simulink library "xpcrealtimedeviceslib"  (Simulink 6.0)
settings: Solver=ode45  SolverMode=SingleTasking  StartTime=0.0  StopTime=10.0  RelTol=1e-3
values from neighbouring files (symbols this model uses):
  baseDec = hex2dec(base(3:end))    [maddiamondmm.m]    (also in maddiamondmm32.m; maddiamondmm32frame.m; maddsmm16at.m; madprometheus.m)
undefined symbols (not defined in the file or in its folder): madrtddm64x0, madrtddm7420, mdartddm6430, mdartddm64x0, mdiortddm64x0, mdiortddm7420, mdirtddm6814, mdortddm6814, mencrtddm6814, misa8255, mpwmrtddm6816, mrtddm6604
libraries: xpcmeasurementcomputinglib x6
settings Model: Creator=adowd  LastModifiedBy=gweast
settings DataIOCC: SignalLoggingName=logsOut
settings OptimizationCC: BooleanDataType=off
settings DebuggingCC: CheckExecutionContextPreStartOutputMsg=on  CheckExecutionContextRuntimeOutputMsg=on  SolverPrmCheckMsg=none
settings HardwareCC: TargetUnknown=on
settings GRTTargetCC: UtilityFuncGeneration=Automatic  LifeSpan=inf
settings SFSimCC: SFSimApplyToAllLibs=on  SFSimBuildMode=Incremental

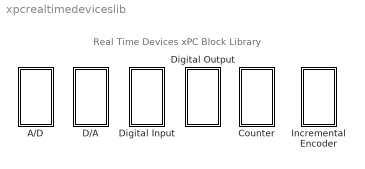
== system xpcrealtimedeviceslib ==
  note: Real Time Devices xPC Block Library
  A/D : Subsystem  EnableExecutionContextPropagation=on
  Counter : Subsystem  EnableExecutionContextPropagation=on
  D/A : Subsystem  EnableExecutionContextPropagation=on
  Digital Input : Subsystem  EnableExecutionContextPropagation=on
  Digital Output : Subsystem  EnableExecutionContextPropagation=on
  Incremental Encoder : Subsystem  EnableExecutionContextPropagation=on

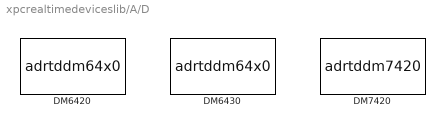
== system xpcrealtimedeviceslib/A/D ==
  "DM6420 " : S-Function  InitFcn=madrtddm64x0(1);  FunctionName=adrtddm64x0  Parameters=channel, coupling, range, gain, ts, baseAddr, boardType  mask(adrtddm6420){channelin=[1], couplingin=[1], rangein=[-10], gainin=[1], ts=0.001, baseAddr=0x300}
      mask prompts: channelin "Channel vector:"; couplingin "Input coupling vector:"; rangein "Range vector:"; gainin "Gain vector:"; ts "Sample time:"; baseAddr "Base address (i.e. 0xd000):"
      mask help:
      | DM6420
      | Real Time Devices
      | Analog Input
      mask init:
      | boardType=1;
      | baseAddr=hex2dec(baseAddr(3:end));
      | channel=0;coupling=0;range=1;gain=0;
      | [channel,coupling,range,gain,maskdisplay,maskdescription]=madrtddm64x0(2, boardType, channelin, couplingin, rangein, gainin);
      | set_param(gcb,'MaskDisplay',maskdisplay);
      | set_param(gcb,'MaskDescription',maskdescription);
      mask Help: helpview(fullfile(docroot, 'mapfiles', 'xpc.map'), 'RealTimeDevices_DM6420_AD')
      mask Display: text(0.05,0.75,'DM6420','horizontalAlignment','left');text(0.05,0.50,'RTD','horizontalAlignment','left');text(0.05,0.25,'AnalogIn','horizontalAlignment','left');port_label('output',1,'1 (SE)');
  "DM6430 " : S-Function  InitFcn=madrtddm64x0(1);  FunctionName=adrtddm64x0  Parameters=channel, coupling, range, gain, ts, baseAddr, boardType  mask(adrtddm6430){channelin=[1], couplingin=[1], gainin=[1], ts=0.001, baseAddr=0x300}
      mask prompts: channelin "Channel vector:"; couplingin "Input coupling vector:"; gainin "Gain vector:"; ts "Sample time:"; baseAddr "Base address (i.e. 0xd000):"
      mask help:
      | DM6430
      | Real Time Devices
      | Analog Input
      mask init:
      | rangein=-10;
      | boardType=2;
      | baseAddr=hex2dec(baseAddr(3:end));
      | channel=0;coupling=0;range=1;gain=0;
      | [channel,coupling,range,gain,maskdisplay,maskdescription]=madrtddm64x0(2, boardType, channelin, couplingin, rangein, gainin);
      | set_param(gcb,'MaskDisplay',maskdisplay);
      | set_param(gcb,'MaskDescription',maskdescription);
      mask Help: helpview(fullfile(docroot, 'mapfiles', 'xpc.map'), 'RealTimeDevices_DM6430_AD')
      mask Display: text(0.05,0.75,'DM6430','horizontalAlignment','left');text(0.05,0.50,'RTD','horizontalAlignment','left');text(0.05,0.25,'AnalogIn','horizontalAlignment','left');port_label('output',1,'1 (SE)');
  "DM7420 " : S-Function  InitFcn=madrtddm7420(1);  FunctionName=adrtddm7420  Parameters=channel, coupling, range, gain, ts, pciSlot, pciDev  mask(adrtddm7420){channelin=[1], couplingin=[1], rangein=[-10], gainin=[1], ts=0.001, pciSlot=-1}
      mask prompts: channelin "Channel vector:"; couplingin "Input coupling vector:"; rangein "Range vector:"; gainin "Gain vector:"; ts "Sample time:"; pciSlot "PCI slot (-1: autosearch):"
      mask help:
      | DM7420
      | Real Time Devices
      | Analog Input
      mask init:
      | pciDev=1;
      | channel=0;coupling=0;range=1;gain=0;
      | [channel,coupling,range,gain,maskdisplay,maskdescription]=madrtddm7420(2, channelin, couplingin, rangein, gainin);
      | set_param(gcb,'MaskDisplay',maskdisplay);
      | set_param(gcb,'MaskDescription',maskdescription);
      mask Help: helpview(fullfile(docroot, 'mapfiles', 'xpc.map'), 'RealTimeDevices_DM7420_AD')
      mask Display: text(0.05,0.75,'DM7420','horizontalAlignment','left');text(0.05,0.50,'RTD','horizontalAlignment','left');text(0.05,0.25,'AnalogIn','horizontalAlignment','left');port_label('output',1,'1 (RSE)');

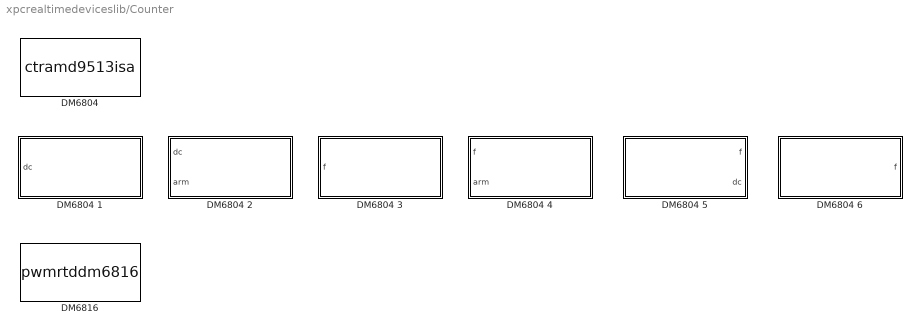
== system xpcrealtimedeviceslib/Counter ==
  "DM6804 " : S-Function  FunctionName=ctramd9513isa  Parameters=io, mm, cms, initir, ir, termir, ts, baseAddress  mask(rtddm6804){mastermode=[], countermode=[], init=[], commands=[], term=[], ts=0.001, baseAddress='0x300'}
      mask prompts: mastermode "Master mode structure:"; countermode "Counter mode structure:"; init "Initialization command structure:"; commands "Runtime command structure:"; term "Termination command structure:"; ts "Sample time:"; baseAddress "9513 chip base address (i.e. 0xd000):"
      mask help:
      | DM6804
      | Real Time Devices
      | AMD9513 Counter
      mask init:
      | baseAddress=hex2dec(baseAddress(3:end));
      | [io,mm, cms, initir, ir, termir]=mamd9513parse(mastermode, countermode, init, commands, term);
      mask Help: helpview(fullfile(docroot, 'mapfiles', 'xpc.map'), 'RealTimeDevices_DM6804_Counter')
      mask Display: disp('AMD9513\nCounter')
  DM6804 1 : Subsystem  EnableExecutionContextPropagation=on  mask(PWM){counterin=1, freq_base=F1=5MHz, freq=0.001, seq=High - Low, level=High, Ts=0.001, baseAddress=0x300}
      mask prompts: counterin "Counter:"; freq_base "Frequency base:"; freq "Relative output frequency:"; seq "Level sequence of square wave:"; level "Level when disarmed:"; Ts "Sample time:"; baseAddress "Base address (i.e. 0xd000):"
      mask help:
      | DM6804
      | Real Time Devices
      | PWM
      mask init:
      | init_arm=0;
      | initduty=0.5;
      | counter=counterin;
      | baseAddress=['0x',dec2hex(hex2dec(baseAddress(3:end))+4)];
      | [MasterMode, CounterMode, Init, Runtime, Term] =pwmarm_amd9513(counter, freq_base, freq, initduty, level, init_arm);
      | level=level-1;
      | seq=seq-1;
      mask Help: helpview(fullfile(docroot, 'mapfiles', 'xpc.map'), 'RealTimeDevices_DM6804-1_Counter')
      mask StyleString: popup(1|2|3|4|5),popup(F1=5MHz|F2=500KHz|F3=50kHz|F4=5kHz|F5=500Hz),edit,popup(High - Low|Low- High),popup(Low|High),edit,edit
      mask Display: text(0.95,0.75,'DM6804','horizontalAlignment','right');text(0.95,0.50,'RTD','horizontalAlignment','right');text(0.95,0.25,'PWM','horizontalAlignment','right');port_label('input',1,[num2str(counterin),' (dc)'] );
  DM6804 2 : Subsystem  EnableExecutionContextPropagation=on  mask(PWM){counterin=1, freq_base=F1=5MHz, freq=0.001, seq=High - Low, level=High, Ts=0.001, baseAddress=0x300}
      mask prompts: counterin "Counter:"; freq_base "Frequency base:"; freq "Relative output frequency:"; seq "Level sequence of square wave:"; level "Level when disarmed:"; Ts "Sample time:"; baseAddress "Base address (i.e. 0xd000):"
      mask help:
      | DM6804
      | Real Time Devices
      | PWM & ARM
      mask init: same as xpcrealtimedeviceslib/Counter/DM6804 1
      mask Help: helpview(fullfile(docroot, 'mapfiles', 'xpc.map'), 'RealTimeDevices_DM6804-2_Counter')
      mask StyleString: popup(1|2|3|4|5),popup(F1=5MHz|F2=500KHz|F3=50kHz|F4=5kHz|F5=500Hz),edit,popup(High - Low|Low- High),popup(Low|High),edit,edit
      mask Display: text(0.95,0.75,'DM6804','horizontalAlignment','right');text(0.95,0.50,'RTD','horizontalAlignment','right');text(0.95,0.25,'PWM & ARM','horizontalAlignment','right');port_label('input',1,[num2str(counterin),' (dc)'] );port_label('input',2,[num2str(counterin),' (arm)'] );
  DM6804 3 : Subsystem  EnableExecutionContextPropagation=on  mask(PWM){counterin=1, freq_base=F1=5MHz, duty=0.001, seq=High - Low, level=High, Ts=0.001, baseAddress=0x300}
      mask prompts: counterin "Counter:"; freq_base "Frequency base:"; duty "Output duty cycle:"; seq "Level sequence of square wave:"; level "Level when disarmed:"; Ts "Sample time:"; baseAddress "Base address (i.e. 0xd000):"
      mask help:
      | DM6804
      | Real Time Devices
      | FM
      mask init:
      | init_arm=0;
      | initfreq=0.005;
      | counter=counterin;
      | baseAddress=['0x',dec2hex(hex2dec(baseAddress(3:end))+4)];
      | [MasterMode, CounterMode, Init, Runtime, Term] =fmarm_amd9513(counter, freq_base, duty, initfreq, level, init_arm);
      | level=level-1;
      | seq=seq-1;
      mask Help: helpview(fullfile(docroot, 'mapfiles', 'xpc.map'), 'RealTimeDevices_DM6804-3_Counter')
      mask StyleString: popup(1|2|3|4|5),popup(F1=5MHz|F2=500KHz|F3=50kHz|F4=5kHz|F5=500Hz),edit,popup(High - Low|Low- High),popup(Low|High),edit,edit
      mask Display: text(0.95,0.75,'DM6804','horizontalAlignment','right');text(0.95,0.50,'RTD','horizontalAlignment','right');text(0.95,0.25,'FM','horizontalAlignment','right');port_label('input',1,[num2str(counterin),' (f)'] );
  DM6804 4 : Subsystem  EnableExecutionContextPropagation=on  mask(FM){counterin=1, freq_base=F1=5MHz, duty=0.001, seq=High - Low, level=High, Ts=0.001, baseAddress=0x300}
      mask prompts: counterin "Counter:"; freq_base "Frequency base:"; duty "Output duty cycle:"; seq "Level sequence of square wave:"; level "Level when disarmed:"; Ts "Sample time:"; baseAddress "Base address (i.e. 0xd000):"
      mask help:
      | DM6804
      | Real Time Devices
      | FM & ARM
      mask init: same as xpcrealtimedeviceslib/Counter/DM6804 3
      mask Help: helpview(fullfile(docroot, 'mapfiles', 'xpc.map'), 'RealTimeDevices_DM6804-4_Counter')
      mask StyleString: popup(1|2|3|4|5),popup(F1=5MHz|F2=500KHz|F3=50kHz|F4=5kHz|F5=500Hz),edit,popup(High - Low|Low- High),popup(Low|High),edit,edit
      mask Display: text(0.95,0.75,'DM6804','horizontalAlignment','right');text(0.95,0.50,'RTD','horizontalAlignment','right');text(0.95,0.25,'FM & ARM','horizontalAlignment','right');port_label('input',1,[num2str(counterin),' (f)'] );port_label('input',2,[num2str(counterin),' (arm)'] );
  DM6804 5 : Subsystem  EnableExecutionContextPropagation=on  mask(PWMcap){counterin=1&2, freq_base=F1=5MHz, Ts=0.001, baseAddress=0x300}
      mask prompts: counterin "Counter:"; freq_base "Frequency base:"; Ts "Sample time:"; baseAddress "Base address (i.e. 0xd000):"
      mask help:
      | DM6804
      | Real Time Devices
      | PWM capture
      mask init:
      | counter=counterin;
      | baseAddress=['0x',dec2hex(hex2dec(baseAddress(3:end))+4)];
      | [MasterMode, CounterMode, Init, Runtime, Term] =pwmcap_amd9513(counter, freq_base);
      mask Help: helpview(fullfile(docroot, 'mapfiles', 'xpc.map'), 'RealTimeDevices_DM6804-5_Counter')
      mask StyleString: popup(1&2|2&3|3&4|4&5),popup(F1=5MHz|F2=500KHz|F3=50kHz|F4=5kHz|F5=500Hz),edit,edit
      mask Display: text(0.05,0.75,'DM6804','horizontalAlignment','left');text(0.05,0.50,'RTD','horizontalAlignment','left');text(0.05,0.25,'PWM capture','horizontalAlignment','left');port_label('output',1,[num2str(counterin),' (f)'] );port_label('output',2,[num2str(counterin+1),' (dc)'] );
  DM6804 6 : Subsystem  EnableExecutionContextPropagation=on  mask(FREQcap){counterin=1, freq_base=F1=5MHz, Ts=0.001, baseAddress=0x300}
      mask prompts: counterin "Counter:"; freq_base "Frequency base:"; Ts "Sample time:"; baseAddress "Base address (i.e. 0xd000):"
      mask help:
      | DM6804
      | Real Time Devices
      | Frquency capture
      mask init:
      | counter=counterin;
      | baseAddress=['0x',dec2hex(hex2dec(baseAddress(3:end))+4)];
      | [MasterMode, CounterMode, Init, Runtime, Term] =freqcap_amd9513(counter, freq_base);
      mask Help: helpview(fullfile(docroot, 'mapfiles', 'xpc.map'), 'RealTimeDevices_DM6804-6_Counter')
      mask StyleString: popup(1|2|3|4|5),popup(F1=5MHz|F2=500KHz|F3=50kHz|F4=5kHz|F5=500Hz),edit,edit
      mask Display: text(0.05,0.75,'DM6804','horizontalAlignment','left');text(0.05,0.50,'RTD','horizontalAlignment','left');text(0.05,0.25,'Freq. capture','horizontalAlignment','left');port_label('output',1,[num2str(counterin),' (f)'] );
  "DM6816 " : S-Function  InitFcn=mpwmrtddm6816(1);  FunctionName=pwmrtddm6816  Parameters=channel, [clock0, clock1, clock2], divisor, sampleTime, baseDec  mask(pwmrtddm6816){channel=[1], clock0=Timer 1 output, clock1=Timer 1 output, clock2=Timer 1 output, divisor=[2, 2, 2], sampleTime=0.001, base=0x300}
      mask prompts: channel "Channel vector:"; clock0 "Clock source for channels 1, 2, 3"; clock1 "Clock source for channels 4, 5, 6"; clock2 "Clock source for channels 7, 8, 9"; divisor "Frequency divisors for timers 0, 1, 2:"; sampleTime "Sample time:"; base "Base address (e.g. 0xd000):"
      mask help:
      | DM6816
      | RTD
      | PWM
      mask init:
      | phase = 2;
      | [maskDisplay, maskDescription, baseDec] = mpwmrtddm6816( phase, channel, divisor, base );
      | set_param(gcb, 'MaskDescription', maskDescription);
      | set_param(gcb, 'MaskDisplay', maskDisplay);
      mask Help: helpview(fullfile(docroot, 'mapfiles', 'xpc.map'), 'RTD_DM6816_PWM')
      mask StyleString: edit,popup(8 MHz clock|Timer 1 output),popup(8 MHz clock|Timer 1 output),popup(8 MHz clock|Timer 1 output),edit,edit,edit
      mask Display: disp('DM6816\nRTD\nPWM'); port_label('input', 1, '1');

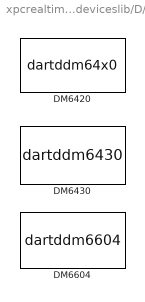
== system xpcrealtimedeviceslib/D/A ==
  "DM6420 " : S-Function  InitFcn=mdartddm64x0(1);  FunctionName=dartddm64x0  Parameters=channel, range, sampletime, baseaddress, boardType  mask(dartddm6420){channel=[1], range=[-5], sampletime=0.001, baseaddress=0x300}
      mask prompts: channel "Channel vector:"; range "Range vector:"; sampletime "Sample time:"; baseaddress "Base address (i.e. 0xd000):"
      mask help:
      | DM6420
      | Real Time Devices
      | Analog Output
      mask init:
      | baseaddress=hex2dec(baseaddress(3:end));
      | boardType=1;
      | [maskdisplay, maskdescription]= mdartddm64x0(2, boardType, channel, range);
      | set_param(gcb,'MaskDisplay',maskdisplay);
      | set_param(gcb,'MaskDescription',maskdescription);
      mask Help: helpview(fullfile(docroot, 'mapfiles', 'xpc.map'), 'RealTimeDevices_DM6420_DA')
      mask Display: text(0.95,0.75,'DM6420','horizontalAlignment','right');text(0.95,0.50,'RTD','horizontalAlignment','right');text(0.95,0.25,'AnalogOut','horizontalAlignment','right');port_label('input',1,'1 (SE)');
  "DM6430 " : S-Function  InitFcn=mdartddm6430(1);  FunctionName=dartddm6430  Parameters=channel, reset, initValue, sampleTime, baseDec  mask(dartddm6430){channel=[1], reset=[1], initValue=[0], sampleTime=.001, base=0x300}
      mask prompts: channel "Channel vector:"; reset "Reset vector:"; initValue "Initial value vector:"; sampleTime "Sample time:"; base "Base address (e.g. 0x300):"
      mask help:
      | DM6430
      | RTD
      | Analog Output
      mask init:
      | phase = 2;
      | [maskDisplay, maskDescription, reset, initValue, baseDec] = mdartddm6430( phase, channel, reset, initValue, base );
      | set_param( gcb, 'MaskDisplay', maskDisplay );
      | set_param( gcb, 'maskDescription', maskDescription );
      mask Help: helpview(fullfile(docroot, 'mapfiles', 'xpc.map'), 'RTD_DM6430_DA')
      mask Display: disp('DM6430\nRTD\nAnalog Output'); port_label('input', 1, '1');
  "DM6604 " : S-Function  InitFcn=mrtddm6604(1);  FunctionName=dartddm6604  Parameters=channel, range, sampletime, baseaddress  mask(dartddm6604){channel=[1], range=[-10], sampletime=0.001, baseaddress=0x300}
      mask prompts: channel "Channel vector:"; range "Range vector:"; sampletime "Sample time:"; baseaddress "Base address (i.e. 0xd000):"
      mask help:
      | Real Time Devices
      | DM6604
      | Analog Output
      mask init:
      | baseaddress=hex2dec(baseaddress(3:end));
      | mrtddm6604(2,channel, range, baseaddress);
      mask Help: helpview(fullfile(docroot, 'mapfiles', 'xpc.map'), 'RealTimeDevices_DM6604_DA')
      mask Display: disp('DM6604\nRTD\nAnalog Output');port_label('input',1,'1');

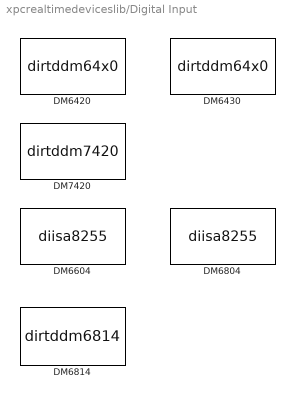
== system xpcrealtimedeviceslib/Digital Input ==
  "DM6420 " : S-Function  InitFcn=mdiortddm64x0(1);  FunctionName=dirtddm64x0  Parameters=channel, port, ts, baseAddr  mask(dirtddm6420){channel=[1], port=0, ts=0.001, baseAddr=0x300}
      mask prompts: channel "Channel vector:"; port "Port (0-1):"; ts "Sample time:"; baseAddr "Base address (i.e. 0xd000):"
      mask help:
      | DM6420
      | RTD
      | Digital Input
      mask init:
      | baseAddr=hex2dec(baseAddr(3:end));
      | type=2;
      | boardType=1;
      | [maskdisplay,maskdescription]=mdiortddm64x0(2, boardType, type, channel, port);
      | set_param(gcb,'MaskDisplay',maskdisplay);
      | set_param(gcb,'MaskDescription',maskdescription);
      mask Help: helpview(fullfile(docroot, 'mapfiles', 'xpc.map'), 'RealTimeDevices_DM6420_DIN')
      mask StyleString: edit,popup(0|1),edit,edit
      mask Display: text(0.05,0.75,'DM6420','horizontalAlignment','left');text(0.05,0.50,'RTD','horizontalAlignment','left');text(0.05,0.25,'DigitalIn','horizontalAlignment','left');port_label('output',1,'1 (P0)');
  "DM6430 " : S-Function  InitFcn=mdiortddm64x0(1);  FunctionName=dirtddm64x0  Parameters=channel, port, ts, baseAddr  mask(dirtddm6430){channel=[1], port=0, ts=0.001, baseAddr=0x300}
      mask prompts: channel "Channel vector:"; port "Port (0-1):"; ts "Sample time:"; baseAddr "Base address (i.e. 0xd000):"
      mask help:
      | DM6430
      | RTD
      | Digital Input
      mask init:
      | baseAddr=hex2dec(baseAddr(3:end));
      | type=2;
      | boardType=2;
      | [maskdisplay,maskdescription]=mdiortddm64x0(2, boardType, type, channel, port);
      | set_param(gcb,'MaskDisplay',maskdisplay);
      | set_param(gcb,'MaskDescription',maskdescription);
      mask Help: helpview(fullfile(docroot, 'mapfiles', 'xpc.map'), 'RealTimeDevices_DM6430_DIN')
      mask StyleString: edit,popup(0|1),edit,edit
      mask Display: text(0.05,0.75,'DM6430','horizontalAlignment','left');text(0.05,0.50,'RTD','horizontalAlignment','left');text(0.05,0.25,'DigitalIn','horizontalAlignment','left');port_label('output',1,'1 (P0)');
  "DM6604 " : S-Function  InitFcn=misa8255(1);  FunctionName=diisa8255  Parameters=channel, port, sampletime, baseaddress, control  mask(dirtddm6604){channel=[1], port=A, chip=1, sampletime=0.001, baseaddress=0x300}
      mask prompts: channel "Channel vector:"; sampletime "Sample time:"; baseaddress "Base address (i.e. 0xd000):"
      mask help:
      | DM6604
      | Real Time Devices
      | Digital Input
      mask init:
      | baseaddress=hex2dec(baseaddress(3:end));
      | control=155;
      | boardType=16;
      | [baseaddress,control,maskdisplay,maskdescription]=misa8255(2, chip, port, channel, baseaddress);
      | set_param(gcb, 'MaskDisplay', maskdisplay);
      | set_param(gcb, 'MaskDescription', maskdescription);
      mask Help: helpview(fullfile(docroot, 'mapfiles', 'xpc.map'), 'RealTimeDevices_DM6604_DIN')
      mask StyleString: edit,popup(A|B|C),popup(1),edit,edit
      mask Display: disp('DM6604\nRTD\nDigital Input');port_label('output',1,'1');
  "DM6804 " : S-Function  InitFcn=misa8255(1);  FunctionName=diisa8255  Parameters=channel, port, sampletime, baseaddress, control  mask(dirtddm6804){channel=[1], port=A, chip=1, sampletime=0.001, baseaddress=0x300}
      mask prompts: channel "Channel vector:"; sampletime "Sample time:"; baseaddress "Base address (i.e. 0xd000):"
      mask help:
      | DM6804
      | Real Time Devices
      | Digital Input
      mask init: same as xpcrealtimedeviceslib/Digital Input/DM6604 
      mask Help: helpview(fullfile(docroot, 'mapfiles', 'xpc.map'), 'RealTimeDevices_DM6804_DIN')
      mask StyleString: edit,popup(A|B|C),popup(1),edit,edit
      mask Display: disp('DM6804\nRTD\nDigital Input');port_label('output',1,'1');
  "DM6814 " : S-Function  InitFcn=mdirtddm6814(1);  FunctionName=dirtddm6814  Parameters=UserData.mode, channel, port, sampleTime, baseDec  mask(dirtddm6814){channel=[1], port=A, sampleTime=.001, baseHex=0x300}
      mask prompts: channel "Channel vector:"; sampleTime "Sample time:"; baseHex "Base address (e.g. 0x300):"
      mask help:
      | DM6814
      | RTD
      | Digital Input
      mask init:
      | phase = 2;
      | [baseDec, maskdisplay, maskdescription] = mdirtddm6814(phase, port, channel, sampleTime, baseHex);
      | UserData = get_param(gcb, 'UserData');
      | set_param(gcb, 'MaskDisplay', maskdisplay);
      | set_param(gcb, 'MaskDescription', maskdescription);
      mask Help: helpview(fullfile(docroot, 'mapfiles', 'xpc.map'), 'RTD_DM6814_DIN')
      mask StyleString: edit,popup(A|B|C),edit,edit
      mask Display: disp('DM6814\nRTD\nDigital Input'); port_label('output', 1, '1');
  "DM7420 " : S-Function  InitFcn=mdiortddm7420(1);  FunctionName=dirtddm7420  Parameters=channel, port, ts, pciSlot, pciDev  mask(dirtddm7420){channel=[1], port=0, ts=0.001, pciSlot=-1}
      mask prompts: channel "Channel vector:"; port "Port (0-1):"; ts "Sample time:"; pciSlot "PCI slot (-1: autosearch):"
      mask help:
      | DM7420
      | RTD
      | Digital Input
      mask init:
      | type=2;
      | pciDev=1;
      | [maskdisplay,maskdescription]=mdiortddm7420(2, type, channel);
      | set_param(gcb,'MaskDisplay',maskdisplay);
      | set_param(gcb,'MaskDescription',maskdescription);
      mask Help: helpview(fullfile(docroot, 'mapfiles', 'xpc.map'), 'RealTimeDevices_DM7420_DIN')
      mask StyleString: edit,popup(0|1),edit,edit
      mask Display: text(0.05,0.75,'DM7420','horizontalAlignment','left');text(0.05,0.50,'RTD','horizontalAlignment','left');text(0.05,0.25,'DigitalIn','horizontalAlignment','left');port_label('output',1,'1');

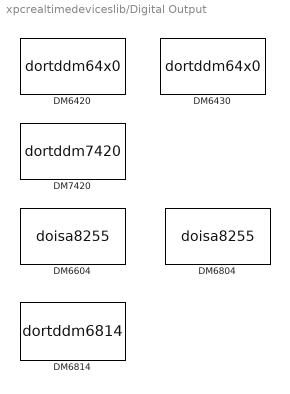
== system xpcrealtimedeviceslib/Digital Output ==
  "DM6420 " : S-Function  InitFcn=mdiortddm64x0(1);  FunctionName=dortddm64x0  Parameters=channel, port, ts, baseAddr  mask(dortddm6420){channel=[1], port=0, ts=0.001, baseAddr=0x300}
      mask prompts: channel "Channel vector:"; port "Port (0-1):"; ts "Sample time:"; baseAddr "Base address (i.e. 0xd000):"
      mask help:
      | DM6420
      | RTD
      | Digital Output
      mask init:
      | baseAddr=hex2dec(baseAddr(3:end));
      | type=1;
      | boardType=1;
      | [maskdisplay,maskdescription]=mdiortddm64x0(2, boardType, type, channel, port);
      | set_param(gcb,'MaskDisplay',maskdisplay);
      | set_param(gcb,'MaskDescription',maskdescription);
      mask Help: helpview(fullfile(docroot, 'mapfiles', 'xpc.map'), 'RealTimeDevices_DM6420_DOUT')
      mask StyleString: edit,popup(0|1),edit,edit
      mask Display: text(0.95,0.75,'DM6420','horizontalAlignment','right');text(0.95,0.50,'RTD','horizontalAlignment','right');text(0.95,0.25,'DigitalOut','horizontalAlignment','right');port_label('input',1,'1 (P0)');
  "DM6430 " : S-Function  InitFcn=mdiortddm64x0(1);  FunctionName=dortddm64x0  Parameters=channel, port, ts, baseAddr  mask(dortddm6430){channel=[1], port=0, ts=0.001, baseAddr=0x300}
      mask prompts: channel "Channel vector:"; port "Port (0-1):"; ts "Sample time:"; baseAddr "Base address (i.e. 0xd000):"
      mask help:
      | DM6430
      | RTD
      | Digital Output
      mask init:
      | baseAddr=hex2dec(baseAddr(3:end));
      | type=1;
      | boardType=2;
      | [maskdisplay,maskdescription]=mdiortddm64x0(2, boardType, type, channel, port);
      | set_param(gcb,'MaskDisplay',maskdisplay);
      | set_param(gcb,'MaskDescription',maskdescription);
      mask Help: helpview(fullfile(docroot, 'mapfiles', 'xpc.map'), 'RealTimeDevices_DM6430_DOUT')
      mask StyleString: edit,popup(0|1),edit,edit
      mask Display: text(0.95,0.75,'DM6430','horizontalAlignment','right');text(0.95,0.50,'RTD','horizontalAlignment','right');text(0.95,0.25,'DigitalOut','horizontalAlignment','right');port_label('input',1,'1 (P0)');
  "DM6604 " : S-Function  InitFcn=misa8255(1);  FunctionName=doisa8255  Parameters=channel, port, reset, initValue, sampletime, baseaddress, control  mask(dortddm6604){channel=[1], port=A, reset=[1], initValue=[0], chip=, sampletime=0.001, baseaddress=0x300}
      mask prompts: channel "Channel vector:"; reset "Reset vector:"; initValue "Initial value vector:"; sampletime "Sample time:"; baseaddress "Base address (e.g. 0xd000):"
      mask help:
      | DM6604
      | Real Time Devices
      | Digital Output
      mask init:
      | baseaddress=hex2dec(baseaddress(3:end));
      | control=155;
      | boardType=16;
      | [baseaddress,control,maskdisplay,maskdescription,reset,initValue]=misa8255(2, chip, port, channel, baseaddress, reset, initValue);
      | set_param(gcb, 'MaskDisplay', maskdisplay);
      | set_param(gcb, 'MaskDescription', maskdescription);
      mask Help: helpview(fullfile(docroot, 'mapfiles', 'xpc.map'), 'RealTimeDevices_DM6604_DOUT')
      mask StyleString: edit,popup(A|B|C),edit,edit,edit,edit,edit
      mask Display: disp('DM6604\nRTD\nDigital Output');port_label('input',1,'1');
  "DM6804 " : S-Function  InitFcn=misa8255(1);  FunctionName=doisa8255  Parameters=channel, port, reset, initValue, sampletime, baseaddress, control  mask(dortddm6804){channel=[1], port=A, reset=[1], initValue=[0], chip=1, sampletime=0.001, baseaddress=0x300}
      mask prompts: channel "Channel vector:"; reset "Reset vector:"; initValue "Initial value vector:"; sampletime "Sample time:"; baseaddress "Base address (e.g. 0xd000):"
      mask help:
      | DM6804
      | Real Time Devices
      | Digital Output
      mask init: same as xpcrealtimedeviceslib/Digital Output/DM6604 
      mask Help: helpview(fullfile(docroot, 'mapfiles', 'xpc.map'), 'RealTimeDevices_DM6804_DOUT')
      mask StyleString: edit,popup(A|B|C),edit,edit,popup(1),edit,edit
      mask Display: disp('DM6804\nRTD\nDigital Output');port_label('input',1,'1');
  "DM6814 " : S-Function  InitFcn=mdortddm6814(1);  FunctionName=dortddm6814  Parameters=UserData.mode, channel, port, reset, initValue, sampleTime, baseDec  mask(dortddm6814){channel=[1], port=A, reset=[1], initValue=[0], sampleTime=.001, baseHex=0x300}
      mask prompts: channel "Channel vector:"; reset "Reset vector:"; initValue "Initial value vector:"; sampleTime "Sample time:"; baseHex "Base address (e.g. 0x300):"
      mask help:
      | DM6814
      | RTD
      | Digital Output
      mask init:
      | phase = 2;
      | [baseDec, maskdisplay, maskdescription] = mdortddm6814(phase, port, channel,  reset, initValue, sampleTime, baseHex);
      | UserData = get_param(gcb, 'UserData');
      | set_param(gcb, 'MaskDisplay', maskdisplay);
      | set_param(gcb, 'MaskDescription', maskdescription);
      mask Help: helpview(fullfile(docroot, 'mapfiles', 'xpc.map'), 'RTD_DM6814_DOUT')
      mask StyleString: edit,popup(A|B|C),edit,edit,edit,edit
      mask Display: disp('DM6814\nRTD\nDigital Output'); port_label('input', 1, '1');
  "DM7420 " : S-Function  InitFcn=mdiortddm7420(1);  FunctionName=dortddm7420  Parameters=channel, port, ts, pciSlot, pciDev  mask(dortddm7420){channel=[1], port=0, ts=0.001, pciSlot=-1}
      mask prompts: channel "Channel vector:"; port "Port (0-1):"; ts "Sample time:"; pciSlot "PCI slot (-1: autosearch):"
      mask help:
      | DM7420
      | RTD
      | Digital Output
      mask init:
      | type=1;
      | pciDev=1;
      | [maskdisplay,maskdescription]=mdiortddm7420(2, type, channel);
      | set_param(gcb,'MaskDisplay',maskdisplay);
      | set_param(gcb,'MaskDescription',maskdescription);
      mask Help: helpview(fullfile(docroot, 'mapfiles', 'xpc.map'), 'RealTimeDevices_DM7420_DOUT')
      mask StyleString: edit,popup(0|1),edit,edit
      mask Display: text(0.95,0.75,'DM7420','horizontalAlignment','right');text(0.95,0.50,'RTD','horizontalAlignment','right');text(0.95,0.25,'DigitalOut','horizontalAlignment','right');port_label('input',1,'1');

== system xpcrealtimedeviceslib/Incremental Encoder ==
  "DM6814 " : S-Function  InitFcn=mencrtddm6814(1);  FunctionName=encrtddm6814  Parameters=UserData.mode, UserData.noDio, channel, initValue, sampleTime, baseDec  mask(encrtddm6814){channel=1, initValue=0, reset=off, sampleTime=0.001, baseHex=0x300}
      mask prompts: initValue "Counter initial value:"; reset "Enable counter reset on px.2 (index input)"; sampleTime "Sample time:"; baseHex "Base address (e.g. 0x300):"
      mask help:
      | DM6814
      | RTD
      | Incremental Encoder
      mask init:
      | phase = 2;
      | [baseDec, maskdisplay, maskdescription] = mencrtddm6814(phase, channel, initValue, reset, sampleTime, baseHex);
      | UserData = get_param(gcb, 'UserData');
      | set_param(gcb, 'MaskDisplay', maskdisplay);
      | set_param(gcb, 'MaskDescription', maskdescription);
      mask Help: helpview(fullfile(docroot, 'mapfiles', 'xpc.map'), 'RealTimeDevices_DM6814_Encoder')
      mask StyleString: popup(1|2|3),edit,checkbox,edit,edit
      mask Display: disp('DM6814\nRTD\nIncremental Encoder'); port_label('output', 1, '1');

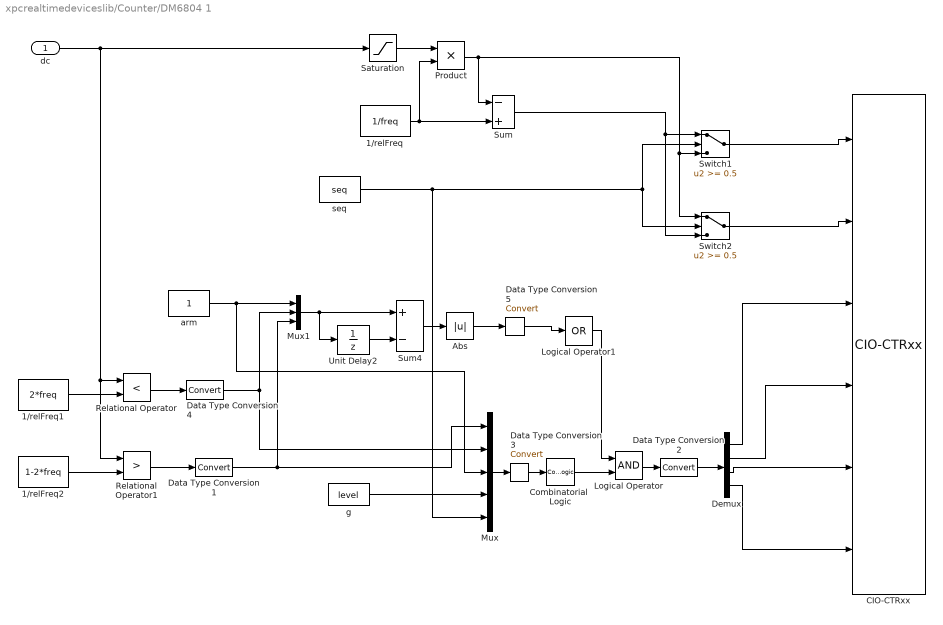
== system xpcrealtimedeviceslib/Counter/DM6804 1 ==
  dc : Inport  LatchInput=off
  1/relFreq : Constant  Value=1/freq
  1/relFreq1 : Constant  Value=2*freq
  1/relFreq2 : Constant  Value=1-2*freq
  Abs : Abs  SaturateOnIntegerOverflow=on
  "CIO-CTRxx " : xpcmeasurementcomputinglib/Counter/CIO-CTRxx   mastermode=MasterMode  countermode=CounterMode  init=Init  commands=Runtime  term=Term  ts=Ts  baseAddress=baseAddress
  Combinatorial  Logic : CombinatorialLogic  TruthTable=[0,0,1,0;0,0,1,0;0,0,0,1;0,0,0,1;0,1,0,0;1,0,0,0;0,1,0,0;1,0,0,0;0,0,1,0;0,0,1,0;0,0,0,1;0,0,0,1;0,0,1,0;0,0,1,0;0,0,1,0;0,0,1,0;0,0,1,0;0,0,1,0;0,0,0,1;0,0,0,1;0,0,0,1;0,0,0,1;0,0,0,1;0,0,0,1;0,0,0,0;0,0,0,0;0,0,0,0;0,0,0,0;0,0,0,0;0,0,0,0;0,0,0,0;0,0,0,0]
  Data Type Conversion1 : DataTypeConversion  OutDataTypeMode=double  SaturateOnIntegerOverflow=on  RndMeth=Zero
  Data Type Conversion2 : DataTypeConversion  SaturateOnIntegerOverflow=on  RndMeth=Zero
  Data Type Conversion3 : DataTypeConversion  SaturateOnIntegerOverflow=on  RndMeth=Zero
  Data Type Conversion4 : DataTypeConversion  OutDataTypeMode=double  SaturateOnIntegerOverflow=on  RndMeth=Zero
  Data Type Conversion5 : DataTypeConversion  SaturateOnIntegerOverflow=on  RndMeth=Zero
  Demux : Demux
  Logical Operator : Logic
  Logical Operator1 : Logic  Operator=OR  Inputs=1
  Mux : Mux  Inputs=5
  Mux1 : Mux  Inputs=3
  Product : Product  SaturateOnIntegerOverflow=on  InputSameDT=on
  Relational Operator : RelationalOperator  Operator=<  InputSameDT=on
  Relational Operator1 : RelationalOperator  Operator=>  InputSameDT=on
  Saturation : Saturate  UpperLimit=1-2*freq  LowerLimit=2*freq  ZeroCross=off
  Sum : Sum  Inputs=-+  SaturateOnIntegerOverflow=on  InputSameDT=on
  Sum4 : Sum  Inputs=+-  SaturateOnIntegerOverflow=on  InputSameDT=on
  Switch1 : Switch  Threshold=0.5  InputSameDT=on
  Switch2 : Switch  Threshold=0.5  InputSameDT=on
  Unit Delay2 : UnitDelay  X0=2  SampleTime=Ts
  arm : Constant
  g : Constant  Value=level
  seq : Constant  Value=seq
  wires:
  Data Type Conversion5/1 -> Logical Operator1/1
  Data Type Conversion3/1 -> Combinatorial  Logic/1
  Data Type Conversion2/1 -> Demux/1
  Data Type Conversion1/1 -> Mux/1, Mux1/3
  Data Type Conversion4/1 -> Mux/2, Mux1/2
  Switch2/1 -> "CIO-CTRxx "/2
  Switch1/1 -> "CIO-CTRxx "/1
  Mux/1 -> Data Type Conversion3/1
  Abs/1 -> Data Type Conversion5/1
  arm/1 -> Mux/3, Mux1/1
  Mux1/1 -> Unit Delay2/1, Sum4/1
  dc/1 -> Relational Operator1/1, Relational Operator/1, Saturation/1
  Saturation/1 -> Product/1
  Sum/1 -> Switch2/3, Switch1/1
  seq/1 -> Mux/5, Switch2/2, Switch1/2
  g/1 -> Mux/4
  Demux/4 -> "CIO-CTRxx "/6
  Demux/3 -> "CIO-CTRxx "/5
  Demux/2 -> "CIO-CTRxx "/4
  Demux/1 -> "CIO-CTRxx "/3
  Logical Operator1/1 -> Logical Operator/1
  Sum4/1 -> Abs/1
  Unit Delay2/1 -> Sum4/2
  Logical Operator/1 -> Data Type Conversion2/1
  Combinatorial  Logic/1 -> Logical Operator/2
  Relational Operator/1 -> Data Type Conversion4/1
  Relational Operator1/1 -> Data Type Conversion1/1
  1/relFreq2/1 -> Relational Operator1/2
  Product/1 -> Switch2/1, Switch1/3, Sum/1
  1/relFreq/1 -> Sum/2, Product/2
  1/relFreq1/1 -> Relational Operator/2

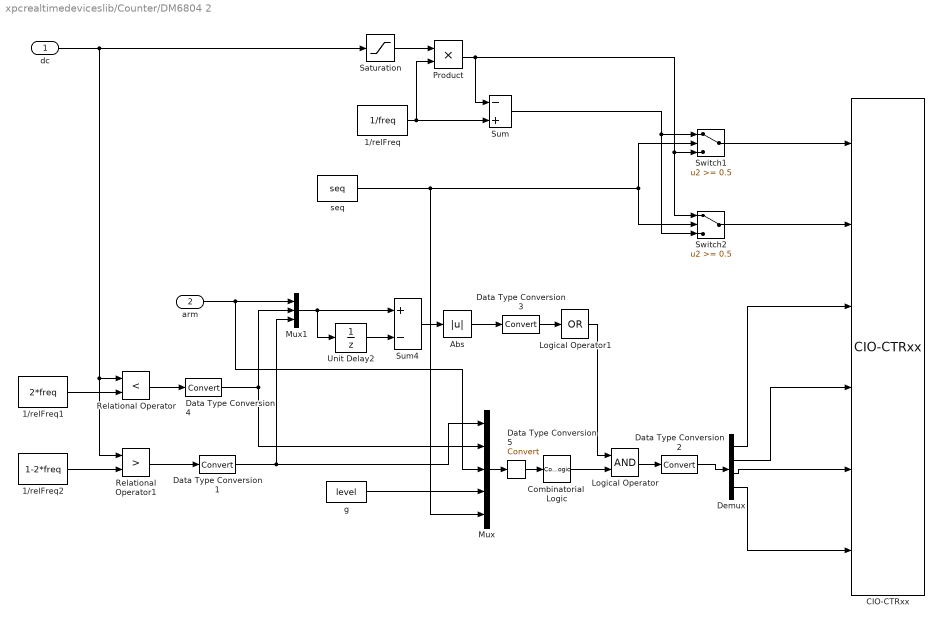
== system xpcrealtimedeviceslib/Counter/DM6804 2 ==
  dc : Inport  LatchInput=off
  arm : Inport  Port=2  LatchInput=off
  1/relFreq : Constant  Value=1/freq
  1/relFreq1 : Constant  Value=2*freq
  1/relFreq2 : Constant  Value=1-2*freq
  Abs : Abs  SaturateOnIntegerOverflow=on
  "CIO-CTRxx " : xpcmeasurementcomputinglib/Counter/CIO-CTRxx   mastermode=MasterMode  countermode=CounterMode  init=Init  commands=Runtime  term=Term  ts=Ts  baseAddress=baseAddress
  Combinatorial  Logic : CombinatorialLogic  TruthTable=[0,0,1,0;0,0,1,0;0,0,0,1;0,0,0,1;0,1,0,0;1,0,0,0;0,1,0,0;1,0,0,0;0,0,1,0;0,0,1,0;0,0,0,1;0,0,0,1;0,0,1,0;0,0,1,0;0,0,1,0;0,0,1,0;0,0,1,0;0,0,1,0;0,0,0,1;0,0,0,1;0,0,0,1;0,0,0,1;0,0,0,1;0,0,0,1;0,0,0,0;0,0,0,0;0,0,0,0;0,0,0,0;0,0,0,0;0,0,0,0;0,0,0,0;0,0,0,0]
  Data Type Conversion1 : DataTypeConversion  OutDataTypeMode=double  SaturateOnIntegerOverflow=on  RndMeth=Zero
  Data Type Conversion2 : DataTypeConversion  SaturateOnIntegerOverflow=on  RndMeth=Zero
  Data Type Conversion3 : DataTypeConversion  SaturateOnIntegerOverflow=on  RndMeth=Zero
  Data Type Conversion4 : DataTypeConversion  OutDataTypeMode=double  SaturateOnIntegerOverflow=on  RndMeth=Zero
  Data Type Conversion5 : DataTypeConversion  SaturateOnIntegerOverflow=on  RndMeth=Zero
  Demux : Demux
  Logical Operator : Logic
  Logical Operator1 : Logic  Operator=OR  Inputs=1
  Mux : Mux  Inputs=5
  Mux1 : Mux  Inputs=3
  Product : Product  SaturateOnIntegerOverflow=on  InputSameDT=on
  Relational Operator : RelationalOperator  Operator=<  InputSameDT=on
  Relational Operator1 : RelationalOperator  Operator=>  InputSameDT=on
  Saturation : Saturate  UpperLimit=1-2*freq  LowerLimit=2*freq  ZeroCross=off
  Sum : Sum  Inputs=-+  SaturateOnIntegerOverflow=on  InputSameDT=on
  Sum4 : Sum  Inputs=+-  SaturateOnIntegerOverflow=on  InputSameDT=on
  Switch1 : Switch  Threshold=0.5  InputSameDT=on
  Switch2 : Switch  Threshold=0.5  InputSameDT=on
  Unit Delay2 : UnitDelay  X0=2  SampleTime=Ts
  g : Constant  Value=level
  seq : Constant  Value=seq
  wires:
  Data Type Conversion5/1 -> Combinatorial  Logic/1
  Data Type Conversion3/1 -> Logical Operator1/1
  Data Type Conversion2/1 -> Demux/1
  Data Type Conversion1/1 -> Mux/1, Mux1/3
  Data Type Conversion4/1 -> Mux/2, Mux1/2
  Switch2/1 -> "CIO-CTRxx "/2
  Switch1/1 -> "CIO-CTRxx "/1
  Mux/1 -> Data Type Conversion5/1
  Abs/1 -> Data Type Conversion3/1
  arm/1 -> Mux/3, Mux1/1
  Mux1/1 -> Unit Delay2/1, Sum4/1
  dc/1 -> Relational Operator1/1, Relational Operator/1, Saturation/1
  Saturation/1 -> Product/1
  Sum/1 -> Switch2/3, Switch1/1
  seq/1 -> Mux/5, Switch2/2, Switch1/2
  g/1 -> Mux/4
  Demux/4 -> "CIO-CTRxx "/6
  Demux/3 -> "CIO-CTRxx "/5
  Demux/2 -> "CIO-CTRxx "/4
  Demux/1 -> "CIO-CTRxx "/3
  Logical Operator1/1 -> Logical Operator/1
  Sum4/1 -> Abs/1
  Unit Delay2/1 -> Sum4/2
  Logical Operator/1 -> Data Type Conversion2/1
  Combinatorial  Logic/1 -> Logical Operator/2
  Relational Operator/1 -> Data Type Conversion4/1
  Relational Operator1/1 -> Data Type Conversion1/1
  1/relFreq2/1 -> Relational Operator1/2
  Product/1 -> Switch2/1, Switch1/3, Sum/1
  1/relFreq/1 -> Sum/2, Product/2
  1/relFreq1/1 -> Relational Operator/2

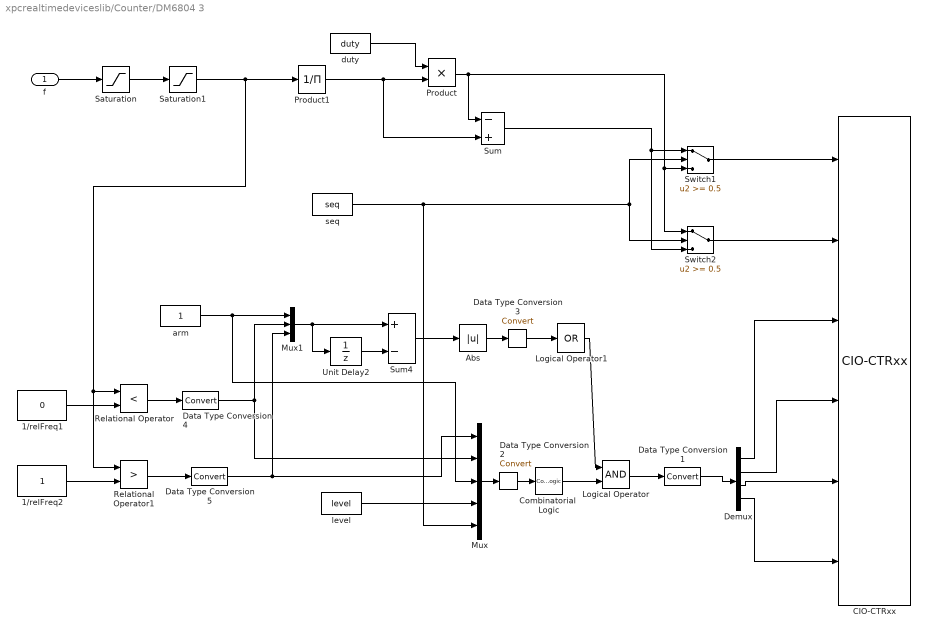
== system xpcrealtimedeviceslib/Counter/DM6804 3 ==
  f : Inport  LatchInput=off
  1/relFreq1 : Constant  Value=0
  1/relFreq2 : Constant
  Abs : Abs  SaturateOnIntegerOverflow=on
  "CIO-CTRxx " : xpcmeasurementcomputinglib/Counter/CIO-CTRxx   mastermode=MasterMode  countermode=CounterMode  init=Init  commands=Runtime  term=Term  ts=Ts  baseAddress=baseAddress
  Combinatorial  Logic : CombinatorialLogic  TruthTable=[0,0,1,0;0,0,1,0;0,0,0,1;0,0,0,1;0,1,0,0;1,0,0,0;0,1,0,0;1,0,0,0;0,0,1,0;0,0,1,0;0,0,0,1;0,0,0,1;0,0,1,0;0,0,1,0;0,0,1,0;0,0,1,0;0,0,1,0;0,0,1,0;0,0,0,1;0,0,0,1;0,0,0,1;0,0,0,1;0,0,0,1;0,0,0,1;0,0,0,0;0,0,0,0;0,0,0,0;0,0,0,0;0,0,0,0;0,0,0,0;0,0,0,0;0,0,0,0]
  Data Type Conversion1 : DataTypeConversion  SaturateOnIntegerOverflow=on  RndMeth=Zero
  Data Type Conversion2 : DataTypeConversion  SaturateOnIntegerOverflow=on  RndMeth=Zero
  Data Type Conversion3 : DataTypeConversion  SaturateOnIntegerOverflow=on  RndMeth=Zero
  Data Type Conversion4 : DataTypeConversion  OutDataTypeMode=double  SaturateOnIntegerOverflow=on  RndMeth=Zero
  Data Type Conversion5 : DataTypeConversion  OutDataTypeMode=double  SaturateOnIntegerOverflow=on  RndMeth=Zero
  Demux : Demux
  Logical Operator : Logic
  Logical Operator1 : Logic  Operator=OR  Inputs=1
  Mux : Mux  Inputs=5
  Mux1 : Mux  Inputs=3
  Product : Product  SaturateOnIntegerOverflow=on  InputSameDT=on
  Product1 : Product  Inputs=/  SaturateOnIntegerOverflow=on  InputSameDT=on
  Relational Operator : RelationalOperator  Operator=<  InputSameDT=on
  Relational Operator1 : RelationalOperator  Operator=>  InputSameDT=on
  Saturation : Saturate  UpperLimit=duty/2  LowerLimit=duty/(2^16-1)  ZeroCross=off
  Saturation1 : Saturate  UpperLimit=(1-duty)/2  LowerLimit=(1-duty)/(2^16-1)  ZeroCross=off
  Sum : Sum  Inputs=-+  SaturateOnIntegerOverflow=on  InputSameDT=on
  Sum4 : Sum  Inputs=+-  SaturateOnIntegerOverflow=on  InputSameDT=on
  Switch1 : Switch  Threshold=0.5  InputSameDT=on
  Switch2 : Switch  Threshold=0.5  InputSameDT=on
  Unit Delay2 : UnitDelay  X0=2  SampleTime=Ts
  arm : Constant
  duty : Constant  Value=duty
  level : Constant  Value=level
  seq : Constant  Value=seq
  wires:
  Data Type Conversion5/1 -> Mux/1, Mux1/3
  Data Type Conversion4/1 -> Mux/2, Mux1/2
  Data Type Conversion3/1 -> Logical Operator1/1
  Data Type Conversion2/1 -> Combinatorial  Logic/1
  Data Type Conversion1/1 -> Demux/1
  Product1/1 -> Sum/2, Product/2
  duty/1 -> Product/1
  Saturation1/1 -> Relational Operator/1, Relational Operator1/1, Product1/1
  Mux/1 -> Data Type Conversion2/1
  Abs/1 -> Data Type Conversion3/1
  arm/1 -> Mux/3, Mux1/1
  Mux1/1 -> Unit Delay2/1, Sum4/1
  f/1 -> Saturation/1
  Saturation/1 -> Saturation1/1
  Sum/1 -> Switch2/3, Switch1/1
  seq/1 -> Mux/5, Switch2/2, Switch1/2
  Switch2/1 -> "CIO-CTRxx "/2
  Switch1/1 -> "CIO-CTRxx "/1
  level/1 -> Mux/4
  Demux/4 -> "CIO-CTRxx "/6
  Demux/3 -> "CIO-CTRxx "/5
  Demux/2 -> "CIO-CTRxx "/4
  Demux/1 -> "CIO-CTRxx "/3
  Logical Operator1/1 -> Logical Operator/1
  Sum4/1 -> Abs/1
  Unit Delay2/1 -> Sum4/2
  Logical Operator/1 -> Data Type Conversion1/1
  Combinatorial  Logic/1 -> Logical Operator/2
  Relational Operator/1 -> Data Type Conversion4/1
  Relational Operator1/1 -> Data Type Conversion5/1
  1/relFreq2/1 -> Relational Operator1/2
  Product/1 -> Switch2/1, Switch1/3, Sum/1
  1/relFreq1/1 -> Relational Operator/2

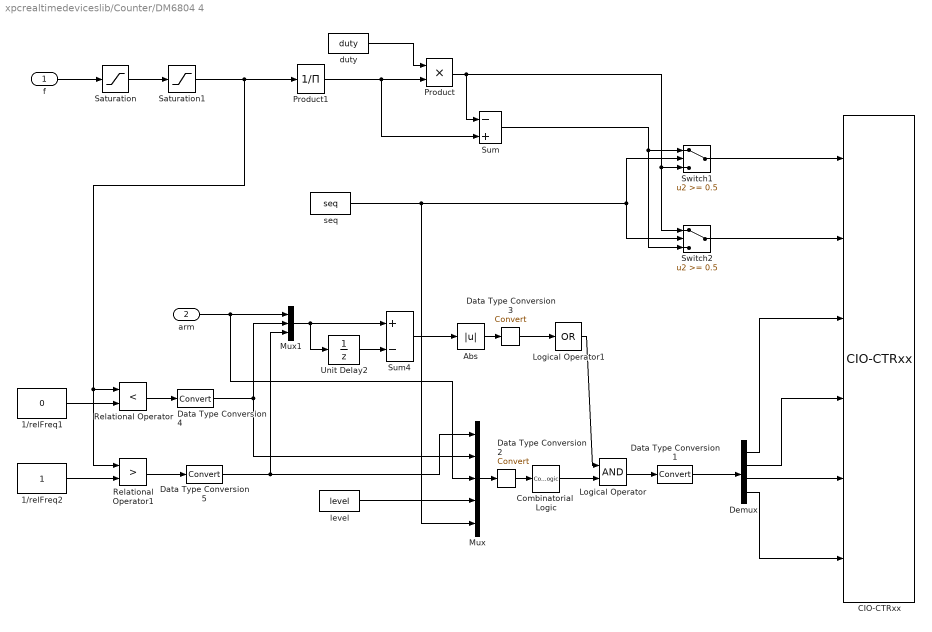
== system xpcrealtimedeviceslib/Counter/DM6804 4 ==
  f : Inport  LatchInput=off
  arm : Inport  Port=2  LatchInput=off
  1/relFreq1 : Constant  Value=0
  1/relFreq2 : Constant
  Abs : Abs  SaturateOnIntegerOverflow=on
  "CIO-CTRxx " : xpcmeasurementcomputinglib/Counter/CIO-CTRxx   mastermode=MasterMode  countermode=CounterMode  init=Init  commands=Runtime  term=Term  ts=Ts  baseAddress=baseAddress
  Combinatorial  Logic : CombinatorialLogic  TruthTable=[0,0,1,0;0,0,1,0;0,0,0,1;0,0,0,1;0,1,0,0;1,0,0,0;0,1,0,0;1,0,0,0;0,0,1,0;0,0,1,0;0,0,0,1;0,0,0,1;0,0,1,0;0,0,1,0;0,0,1,0;0,0,1,0;0,0,1,0;0,0,1,0;0,0,0,1;0,0,0,1;0,0,0,1;0,0,0,1;0,0,0,1;0,0,0,1;0,0,0,0;0,0,0,0;0,0,0,0;0,0,0,0;0,0,0,0;0,0,0,0;0,0,0,0;0,0,0,0]
  Data Type Conversion1 : DataTypeConversion  SaturateOnIntegerOverflow=on  RndMeth=Zero
  Data Type Conversion2 : DataTypeConversion  SaturateOnIntegerOverflow=on  RndMeth=Zero
  Data Type Conversion3 : DataTypeConversion  SaturateOnIntegerOverflow=on  RndMeth=Zero
  Data Type Conversion4 : DataTypeConversion  OutDataTypeMode=double  SaturateOnIntegerOverflow=on  RndMeth=Zero
  Data Type Conversion5 : DataTypeConversion  OutDataTypeMode=double  SaturateOnIntegerOverflow=on  RndMeth=Zero
  Demux : Demux
  Logical Operator : Logic
  Logical Operator1 : Logic  Operator=OR  Inputs=1
  Mux : Mux  Inputs=5
  Mux1 : Mux  Inputs=3
  Product : Product  SaturateOnIntegerOverflow=on  InputSameDT=on
  Product1 : Product  Inputs=/  SaturateOnIntegerOverflow=on  InputSameDT=on
  Relational Operator : RelationalOperator  Operator=<  InputSameDT=on
  Relational Operator1 : RelationalOperator  Operator=>  InputSameDT=on
  Saturation : Saturate  UpperLimit=duty/2  LowerLimit=duty/(2^16-1)  ZeroCross=off
  Saturation1 : Saturate  UpperLimit=(1-duty)/2  LowerLimit=(1-duty)/(2^16-1)  ZeroCross=off
  Sum : Sum  Inputs=-+  SaturateOnIntegerOverflow=on  InputSameDT=on
  Sum4 : Sum  Inputs=+-  SaturateOnIntegerOverflow=on  InputSameDT=on
  Switch1 : Switch  Threshold=0.5  InputSameDT=on
  Switch2 : Switch  Threshold=0.5  InputSameDT=on
  Unit Delay2 : UnitDelay  X0=2  SampleTime=Ts
  duty : Constant  Value=duty
  level : Constant  Value=level
  seq : Constant  Value=seq
  wires:
  Data Type Conversion5/1 -> Mux/1, Mux1/3
  Data Type Conversion4/1 -> Mux/2, Mux1/2
  Data Type Conversion3/1 -> Logical Operator1/1
  Data Type Conversion2/1 -> Combinatorial  Logic/1
  Data Type Conversion1/1 -> Demux/1
  Product1/1 -> Sum/2, Product/2
  duty/1 -> Product/1
  Saturation1/1 -> Relational Operator/1, Relational Operator1/1, Product1/1
  Mux/1 -> Data Type Conversion2/1
  Abs/1 -> Data Type Conversion3/1
  arm/1 -> Mux/3, Mux1/1
  Mux1/1 -> Unit Delay2/1, Sum4/1
  f/1 -> Saturation/1
  Saturation/1 -> Saturation1/1
  Sum/1 -> Switch2/3, Switch1/1
  seq/1 -> Mux/5, Switch2/2, Switch1/2
  Switch2/1 -> "CIO-CTRxx "/2
  Switch1/1 -> "CIO-CTRxx "/1
  level/1 -> Mux/4
  Demux/4 -> "CIO-CTRxx "/6
  Demux/3 -> "CIO-CTRxx "/5
  Demux/2 -> "CIO-CTRxx "/4
  Demux/1 -> "CIO-CTRxx "/3
  Logical Operator1/1 -> Logical Operator/1
  Sum4/1 -> Abs/1
  Unit Delay2/1 -> Sum4/2
  Logical Operator/1 -> Data Type Conversion1/1
  Combinatorial  Logic/1 -> Logical Operator/2
  Relational Operator/1 -> Data Type Conversion4/1
  Relational Operator1/1 -> Data Type Conversion5/1
  1/relFreq2/1 -> Relational Operator1/2
  Product/1 -> Switch2/1, Switch1/3, Sum/1
  1/relFreq1/1 -> Relational Operator/2

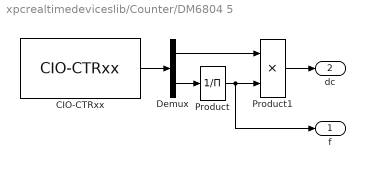
== system xpcrealtimedeviceslib/Counter/DM6804 5 ==
  "CIO-CTRxx " : xpcmeasurementcomputinglib/Counter/CIO-CTRxx   mastermode=MasterMode  countermode=CounterMode  init=Init  commands=Runtime  term=Term  ts=Ts  baseAddress=baseAddress
  Demux : Demux  Outputs=2
  Product : Product  Inputs=/  SaturateOnIntegerOverflow=on  InputSameDT=on
  Product1 : Product  Inputs=**  SaturateOnIntegerOverflow=on  InputSameDT=on
  f : Outport
  dc : Outport  Port=2
  wires:
  Product1/1 -> dc/1
  Product/1 -> Product1/2, f/1
  Demux/2 -> Product/1
  Demux/1 -> Product1/1
  "CIO-CTRxx "/1 -> Demux/1

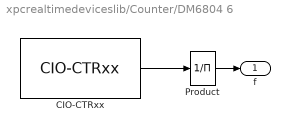
== system xpcrealtimedeviceslib/Counter/DM6804 6 ==
  "CIO-CTRxx " : xpcmeasurementcomputinglib/Counter/CIO-CTRxx   mastermode=MasterMode  countermode=CounterMode  init=Init  commands=Runtime  term=Term  ts=Ts  baseAddress=baseAddress
  Product : Product  Inputs=/  SaturateOnIntegerOverflow=on  InputSameDT=on
  f : Outport
  wires:
  Product/1 -> f/1
  "CIO-CTRxx "/1 -> Product/1
